simulink model "Simulink_Tutorial"  (R2021b)
settings: Solver=FixedStepAuto  StartTime=0.0  StopTime=100  FixedStep=0.01  RelTol=1e-3
settings Model: Creator=basti  LastModifiedBy=basti

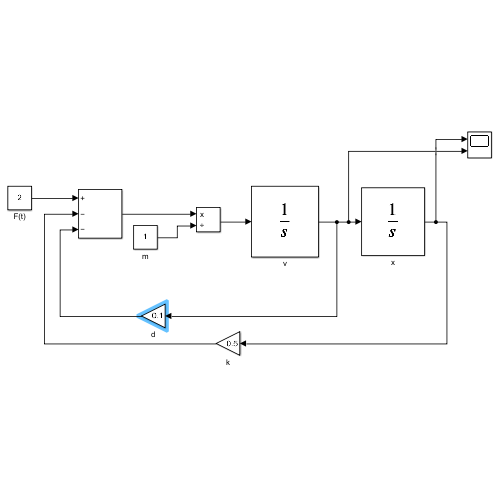
[thumbnail: Simulink's stored preview of the top-level diagram]
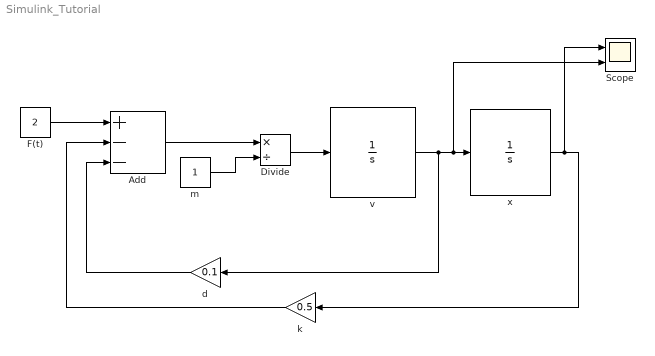
== system Simulink_Tutorial ==
  Add : Sum  Inputs=+--
  Divide : Product  Inputs=*/
  F(t) : Constant  Value=2
  Scope : Scope  NumInputPorts=2
  d : Gain  Gain=0.1
  k : Gain  Gain=0.5
  m : Constant
  v : Integrator
  x : Integrator  InitialCondition=-10
  wires:
  v/1 -> Scope/2, x/1, d/1
  F(t)/1 -> Add/1
  x/1 -> Scope/1, k/1
  d/1 -> Add/3
  k/1 -> Add/2
  Divide/1 -> v/1
  m/1 -> Divide/2
  Add/1 -> Divide/1
